simulink model "Ejercicio4RLCVoltaje"  (R2021b)
settings: Solver=VariableStepAuto  StartTime=0.0  StopTime=300.0  RelTol=1e-3
settings Model: Creator=startupole  LastModifiedBy=startupole

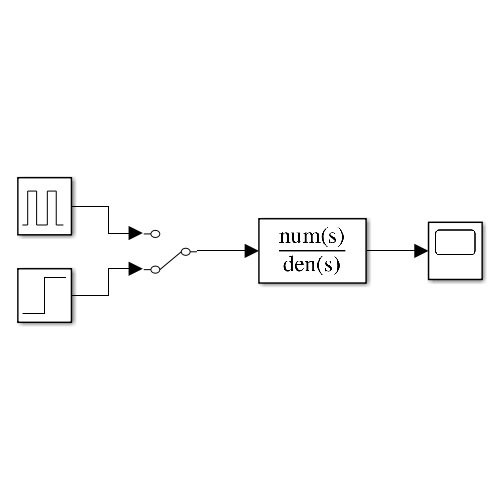
[thumbnail: Simulink's stored preview of the top-level diagram]
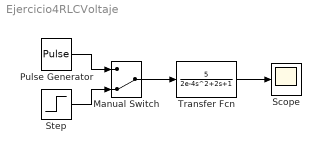
== system Ejercicio4RLCVoltaje ==
  Manual Switch : ManualSwitch  CurrentSetting=0
  Pulse Generator : DiscretePulseGenerator  PulseType=Time based  Period=10  PulseWidth=5
  Scope : Scope
  Step : Step  SampleTime=0
  Transfer Fcn : TransferFcn  Numerator=[5]  Denominator=[2e-4 2 1]
  wires:
  Pulse Generator/1 -> Manual Switch/1
  Step/1 -> Manual Switch/2
  Manual Switch/1 -> Transfer Fcn/1
  Transfer Fcn/1 -> Scope/1
